simulink subsystem "Propulsion_Subsystem"  (R2026a)
settings: Solver=VariableStepAuto
settings Model: Creator=Eeman Aleem  LastModifiedBy=Eeman Aleem

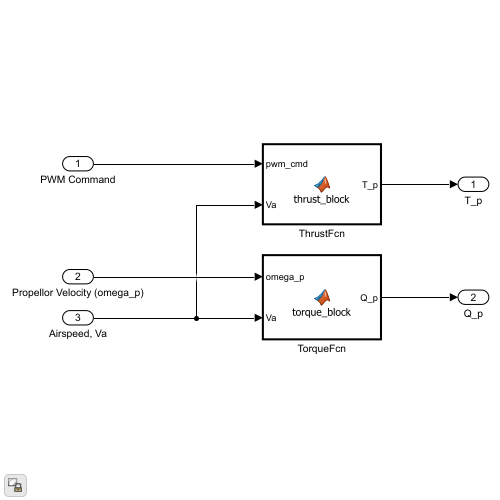
[thumbnail: Simulink's stored preview of the top-level diagram]
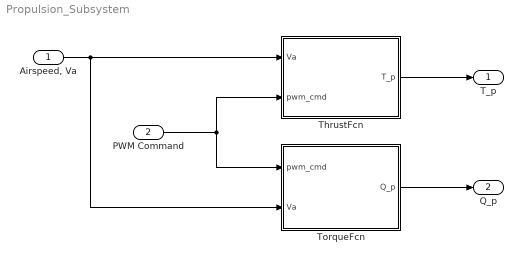
== system Propulsion_Subsystem ==
  "Airspeed, Va" : Inport
  PWM Command : Inport  Port=2
  ThrustFcn : MATLAB Function  TreatAsAtomicUnit=on
  TorqueFcn : MATLAB Function  TreatAsAtomicUnit=on
  T_p : Outport
  Q_p : Outport  Port=2
  wires:
  ThrustFcn/1(T_p) -> T_p/1
  TorqueFcn/1(Q_p) -> Q_p/1
  PWM Command/1 -> TorqueFcn/1(pwm_cmd), ThrustFcn/2(pwm_cmd)
  "Airspeed, Va"/1 -> TorqueFcn/2(Va), ThrustFcn/1(Va)

== matlab function Propulsion_Subsystem/ThrustFcn ==
  data: T_p output; Va input; pwm_cmd input
function T_p = thrust_block(Va, pwm_cmd)
    rho = GeoConsts.rho; 
    S_prop = GeoConsts.S_prop;
    C_prop = GeoConsts.C_prop;
    k_motor = LateralCoeffs.k_motor;
    
    % Thrust force (along x-axis of body frame)
    % From Pg. 53 of Small Unmanned Aircraft: Theory & Practice
    thrust_force = (1/2) * rho * S_prop * C_prop * ((k_motor * pwm_cmd)^2 - (Va^2))
    T_p = [thrust_force, 0, 0];
end

== matlab function Propulsion_Subsystem/TorqueFcn ==
  data: pwm_cmd input; Q_p output; Va input
function Q_p = torque_block(pwm_cmd, Va)
    k_Tp = LateralCoeffs.k_Tp;
    k_omega = LateralCoeffs.k_omega;

    torque = -1 * k_Tp * (k_omega * pwm_cmd)^2;
    Q_p = [torque, 0, 0];
end
